simulink model "original_model2"  (R2016b)
settings: Solver=FixedStepAuto  StartTime=0.0  StopTime=1  FixedStep=0.02  RelTol=1e-3
values from neighbouring files (symbols this model uses):
  rho = [rho1 rho2 rho3 rho4]    [leastSquare.m]    (also in leastSquare2.m = (transpose(A)*A)\transpose(A)*b; parameters.mat = [-1.71136748701 2.88809791639 8.34085809492 -3.97806529373])
  sig = (transpose(A)*A)\transpose(A)*b    [leastSquare.m]    (also in leastSquare2.m; parameters.mat = [11.0155519472 -6.53364462652 33.0155389324 0.441275229296 1)
settings Model: Creator=Ernie  LastModifiedBy=Ernie

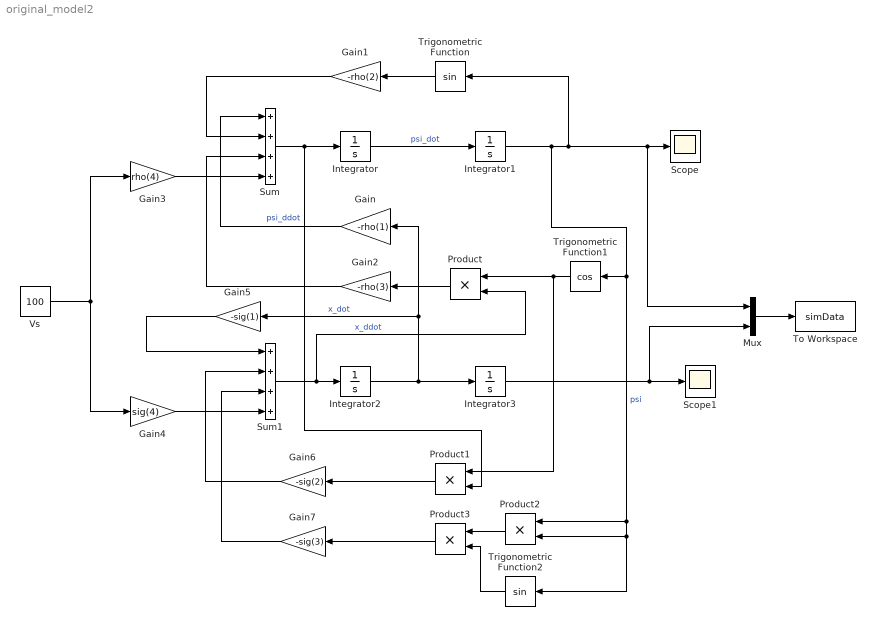
== system original_model2 ==
  Gain : Gain  Gain=-rho(1)
  Gain1 : Gain  Gain=-rho(2)
  Gain2 : Gain  Gain=-rho(3)
  Gain3 : Gain  Gain=rho(4)
  Gain4 : Gain  Gain=sig(4)
  Gain5 : Gain  Gain=-sig(1)
  Gain6 : Gain  Gain=-sig(2)
  Gain7 : Gain  Gain=-sig(3)
  Integrator{,1..3} (4 alike) : Integrator
  Mux : Mux  Inputs=2
  Product{,1..3} (4 alike) : Product
  Scope : Scope
  Scope1 : Scope
  Sum : Sum  Inputs=++++
  Sum1 : Sum  Inputs=++++
  To Workspace : ToWorkspace  VariableName=simData  SaveFormat=Timeseries  SampleTime=-1
  Trigonometric Function : Trigonometry
  Trigonometric Function1 : Trigonometry  Operator=cos
  Trigonometric Function2 : Trigonometry
  Vs : Constant  Value=100
  wires:
  Integrator/1 -> Integrator1/1  "psi_dot"
  Integrator2/1 -> Gain5/1, Gain/1, Integrator3/1  "x_dot"
  Sum1/1 -> Product/2, Integrator2/1  "x_ddot"
  Sum/1 -> Product1/2, Integrator/1  "psi_ddot"
  Gain/1 -> Sum/1
  Trigonometric Function/1 -> Gain1/1
  Integrator1/1 -> Trigonometric Function2/1, Product2/2, Product2/1, Trigonometric Function1/1, Mux/1, Scope/1, Trigonometric Function/1  "psi"
  Gain1/1 -> Sum/2
  Product/1 -> Gain2/1
  Trigonometric Function1/1 -> Product1/1, Product/1
  Gain2/1 -> Sum/3
  Gain3/1 -> Sum/4
  Vs/1 -> Gain4/1, Gain3/1
  Gain4/1 -> Sum1/4
  Gain5/1 -> Sum1/1
  Product1/1 -> Gain6/1
  Gain6/1 -> Sum1/2
  Product2/1 -> Product3/1
  Trigonometric Function2/1 -> Product3/2
  Product3/1 -> Gain7/1
  Gain7/1 -> Sum1/3
  Integrator3/1 -> Mux/2, Scope1/1
  Mux/1 -> To Workspace/1
